simulink model "s1"  (R2016a)
settings: Solver=VariableStepAuto  SolverMode=SingleTasking  StartTime=0.0  StopTime=10.0  RelTol=1e-3
libraries: simulink x1
settings Model: Creator=10973  LastModifiedBy=10973
settings DataIOCC: LimitDataPoints=on  SaveOutput=off  SaveTime=off
settings OptimizationCC: BlockReduction=off  BooleanDataType=off
settings DebuggingCC: SaveWithParameterizedLinksMsg=none  UnderspecifiedInitializationDetection=Classic  MergeDetectMultiDrivingBlocksExec=none  SignalResolutionControl=TryResolveAllWithWarning  AllowSymbolicDim=off
settings HardwareCC: TargetUnknown=on

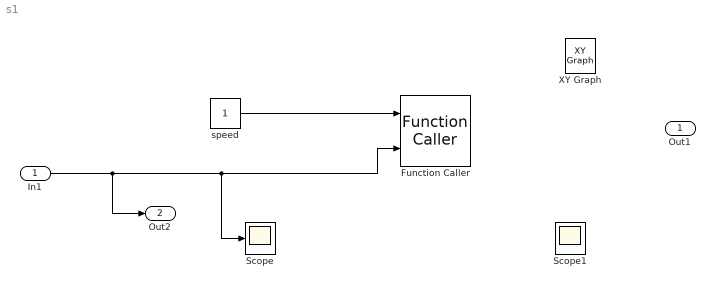
== system s1 ==
  In1 : Inport
  Function Caller : FunctionCaller  FunctionPrototype=y = f(v,gamma)
  Scope : Scope
  Scope1 : Scope
  XY Graph : simulink/Sinks/XY Graph  xmin=-1  xmax=1  ymin=-1  ymax=1  st=-1
  speed : Constant
  Out1 : Outport
  Out2 : Outport  Port=2
  wires:
  speed/1 -> Function Caller/1
  In1/1 -> Function Caller/2, Scope/1, Out2/1
  ? -> XY Graph/1
